simulink model "uC_code"  (R2018b)
settings: Solver=FixedStepDiscrete  StartTime=0.0  StopTime=inf  RelTol=1e-3
PreLoadFcn:
  | LQR_control_design
values from neighbouring files (symbols this model uses):
  ADC_bits = 12    [LQR_control_design.m]    (also in UserSettings.m)
  ADC_Vref = 3.3    [LQR_control_design.m]    (also in UserSettings.m)
  current_gain = 0.5    [LQR_control_design.m]    (also in UserSettings.m)
  current_offset = 1    [LQR_control_design.m]    (also in UserSettings.m)
  K = -K    (= -0.383)    [LQG_control_design.m]    (also in LQR_control_design.m = -(1/R).*B'*Sinf; myLQR.m = -(1/R).*B'*Sinf; myREF.m = [Kw Ki])
  omega_gain = 0.5    [LQR_control_design.m]    (also in UserSettings.m)
  omega_offset = 1    [LQR_control_design.m]    (also in UserSettings.m)
  PPR = 1000    [LQR_control_design.m]    (also in UserSettings.m)
  Vact = 12    [LQR_control_design.m]
undefined symbols (not defined in the file or in its folder): DiscIntNeverNeededParam
libraries: mbedblockslib x5, powerlib_meascontrol x2, dspswit3 x1, discretizing x1
settings Model: ExtModeTrigDuration=10  Creator=angel  LastModifiedBy=angel
settings OptimizationCC: DefaultParameterBehavior=Inlined  UseDivisionForNetSlopeComputation=on  UseFloatMulNetSlope=on  UseSpecifiedMinMax=on  InlineInvariantSignals=on  EnhancedBackFolding=on  BooleansAsBitfields=on  PassReuseOutputArgsAs=Individual arguments  StateBitsets=on  DataBitsets=on  ZeroExternalMemoryAtStartup=off  ZeroInternalMemoryAtStartup=off  NoFixptDivByZeroProtection=on  EfficientFloat2IntCast=on  LifeSpan=1  MaxStackSize=64  OptimizeBlockOrder=speed  DifferentSizesBufferReuse=on
settings DebuggingCC: SignalInfNanChecking=error  IntegerOverflowMsg=error  ParameterTunabilityLossMsg=error  AssertControl=DisableAll  SFUndirectedBroadcastEventsDiag=error
settings HardwareCC: ProdBitPerPointer=32  ProdBitPerSizeT=32  ProdBitPerPtrDiffT=32  ProdLargestAtomicInteger=Long  ProdLargestAtomicFloat=Double  ProdWordSize=32  ProdLongLongMode=on  ProdHWDeviceType=ARM Compatible->ARM Cortex
settings SFSimCC: CompileTimeRecursionLimit=0  EnableRuntimeRecursion=off  MATLABDynamicMemAlloc=off
settings RTWCC: SystemTargetFile=ert.tlc  HardwareBoard=STM32 Nucleo F411RE  TemplateMakefile=ert_default_tmf  GenerateReport=on  Toolchain=GNU Tools for ARM Embedded Processors  BuildConfiguration=Faster Runs  IncludeHyperlinkInReport=on  LaunchReport=on  GenerateTraceInfo=on  GenerateTraceReport=on  GenerateTraceReportSl=on  GenerateTraceReportSf=on  GenerateTraceReportEml=on  GenerateCodeMetricsReport=on
settings CodeAppCC: ForceParamTrailComments=on  IgnoreCustomStorageClasses=off  OperatorAnnotations=on  SimulinkDataObjDesc=on  SFDataObjDesc=on  CustomSymbolStrGlobalVar=rt$N$M  CustomSymbolStrType=$N$M  CustomSymbolStrFcn=$N$M$F  CustomSymbolStrMacro=$N$M  InsertBlockDesc=on
settings ERTTargetCC: UtilityFuncGeneration=Shared location  IncludeMdlTerminateFcn=off  CombineSignalStateStructs=on  SupportAbsoluteTime=off  SupportComplex=off  SupportNonInlinedSFcns=on  ParenthesesLevel=Maximum  CastingMode=Standards  GenerateSharedConstants=off  InlinedParameterPlacement=NonHierarchical  ERTFilePackagingFormat=CompactWithDataFile  EnableSignedLeftShifts=off  EnableSignedRightShifts=off

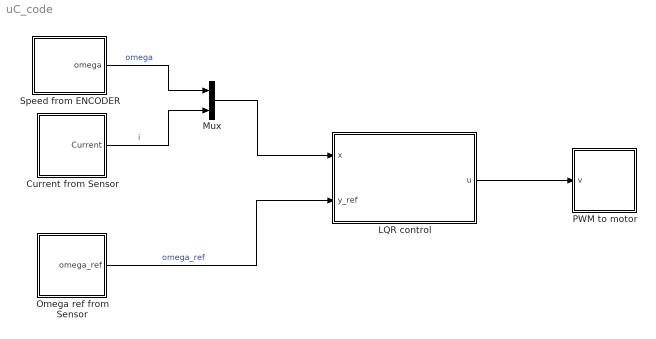
== system uC_code ==
  Current from Sensor : Subsystem
      mask Display: image('E:\Università\Magistrale - Advanced Automotive Electronic Engineering\Compliance Design of Automotive Systems\motor-control\MATLAB\images\lowres-INFIN_Icon_Current_02.eps.png');
  LQR control : Subsystem
  Mux : Mux  Inputs=2
  Omega ref from Sensor : Subsystem
      mask Display: image('E:\Università\Magistrale - Advanced Automotive Electronic Engineering\Compliance Design of Automotive Systems\motor-control\MATLAB\images\65193.png');
  PWM to motor : Subsystem
      mask Display: image('E:\Università\Magistrale - Advanced Automotive Electronic Engineering\Compliance Design of Automotive Systems\motor-control\MATLAB\images\PWM-Icon.png');
  Speed from ENCODER : Subsystem
      mask Display: image('E:\Università\Magistrale - Advanced Automotive Electronic Engineering\Compliance Design of Automotive Systems\motor-control\MATLAB\images\Cattura.JPG');
  wires:
  Speed from ENCODER/1(omega) -> Mux/1  "omega"
  Current from Sensor/1(Current) -> Mux/2  "i"
  Mux/1 -> LQR control/1(x)
  LQR control/1(u) -> PWM to motor/1(v)
  Omega ref from Sensor/1(omega_ref) -> LQR control/2(y_ref)  "omega_ref"

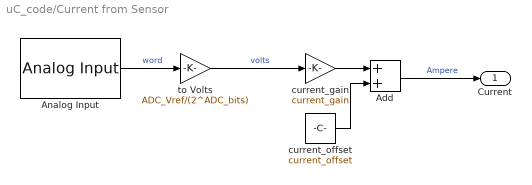
== system uC_code/Current from Sensor ==
  Add : Sum
  Analog Input : mbedblockslib/Analog Input  Pin=PB_0  ReadResultsOnly=off  ConversionTriggerSource=Software  ExternalTriggerType=uint32( 0 )  OutputDataType=double  EnableConversionCompleteNotify=off  EnableOuputStatus=off  SampleTime=-1
      settings: SourceProductName=Simulink Coder Support Package for BBC microbit Board  SourceProductBaseCode=MICROBIT
  current_gain : Gain  Gain=current_gain
  current_offset : Constant  Value=current_offset
  to Volts : Gain  Gain=ADC_Vref/(2^ADC_bits)
  Current : Outport
  wires:
  Analog Input/1 -> to Volts/1  "word"
  current_gain/1 -> Add/1
  current_offset/1 -> Add/2
  to Volts/1 -> current_gain/1  "volts"
  Add/1 -> Current/1  "Ampere"

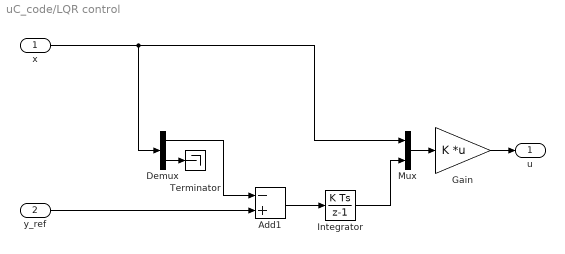
== system uC_code/LQR control ==
  x : Inport
  y_ref : Inport  Port=2
  Add1 : Sum  Inputs=-+
  Demux : Demux  Outputs=2
  Gain : Gain  Gain=K  Multiplication=Matrix(K*u) (u vector)
  Integrator : DiscreteIntegrator  SampleTime=1.0  ICPrevOutput=DiscIntNeverNeededParam  ICPrevScaledInput=DiscIntNeverNeededParam  mask(DiscretizedDiscreteIntegrator){}
      mask init:
      | %zoh
  Mux : Mux  Inputs=2
  Terminator : Terminator
  u : Outport
  wires:
  Mux/1 -> Gain/1
  Demux/1 -> Add1/1
  y_ref/1 -> Add1/2
  Gain/1 -> u/1
  Integrator/1 -> Mux/2
  Add1/1 -> Integrator/1
  x/1 -> Mux/1, Demux/1
  Demux/2 -> Terminator/1

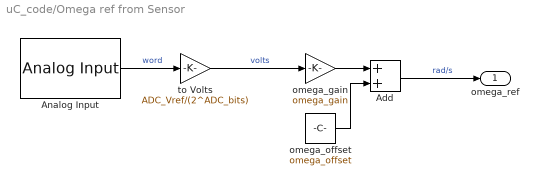
== system uC_code/Omega ref from Sensor ==
  Add : Sum
  Analog Input : mbedblockslib/Analog Input  Pin=PC_0  ReadResultsOnly=off  ConversionTriggerSource=Software  ExternalTriggerType=uint32( 0 )  OutputDataType=double  EnableConversionCompleteNotify=off  EnableOuputStatus=off  SampleTime=-1
      settings: SourceProductName=Simulink Coder Support Package for BBC microbit Board  SourceProductBaseCode=MICROBIT
  omega_gain : Gain  Gain=omega_gain
  omega_offset : Constant  Value=omega_offset
  to Volts : Gain  Gain=ADC_Vref/(2^ADC_bits)
  omega_ref : Outport
  wires:
  Add/1 -> omega_ref/1  "rad/s"
  to Volts/1 -> omega_gain/1  "volts"
  omega_offset/1 -> Add/2
  omega_gain/1 -> Add/1
  Analog Input/1 -> to Volts/1  "word"

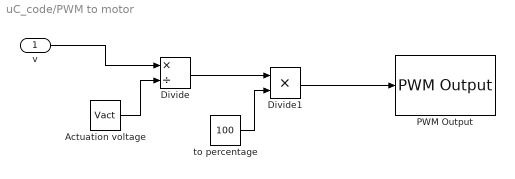
== system uC_code/PWM to motor ==
  v : Inport
  Actuation voltage : Constant  Value=Vact
  Divide : Product  Inputs=*/
  Divide1 : Product  Inputs=**
  PWM Output : mbedblockslib/PWM Output  Pin=PA_3  EnableInputFrequency=off  InitialFrequency=2000  InitialDutyCycle=50  NotificationType=None
      settings: SourceProductName=Simulink Coder Support Package for BBC microbit Board  SourceProductBaseCode=MICROBIT
  to percentage : Constant  Value=100
  wires:
  Actuation voltage/1 -> Divide/2
  v/1 -> Divide/1
  Divide/1 -> Divide1/1
  to percentage/1 -> Divide1/2
  Divide1/1 -> PWM Output/1

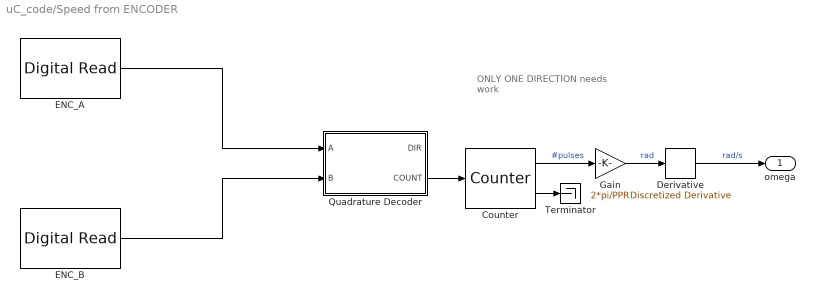
== system uC_code/Speed from ENCODER ==
  note: ONLY ONE DIRECTION
      | needs work
  Counter : dspswit3/Counter  Direction=Up  CountEvent=Rising edge  CounterSize=User defined  MaxCount=255  InitialCount=0  Output=Count and Hit  HitValue=32  ResetInput=off  SamplesPerFrame=1  Ts=1  CntDtype=double  HitDtype=Logical
  Derivative : discretizing/Discretized Derivative  method=tustin  SampleTime=1.0  Wc=1
  ENC_A : mbedblockslib/Digital Read  Pin=PA_0  Direction=input  SampleTime=-1
      settings: SourceProductName=Simulink Coder Support Package for BBC microbit Board  SourceProductBaseCode=MICROBIT
  ENC_B : mbedblockslib/Digital Read  Pin=PA_1  Direction=input  SampleTime=-1
      settings: SourceProductName=Simulink Coder Support Package for BBC microbit Board  SourceProductBaseCode=MICROBIT
  Gain : Gain  Gain=2*pi/PPR
  Quadrature Decoder : Subsystem
  Terminator : Terminator
  omega : Outport
  wires:
  ENC_A/1 -> Quadrature Decoder/1(A)
  ENC_B/1 -> Quadrature Decoder/2(B)
  Quadrature Decoder/2(COUNT) -> Counter/1
  Counter/1 -> Gain/1  "#pulses"
  Gain/1 -> Derivative/1  "rad"
  Derivative/1 -> omega/1  "rad/s"
  Counter/2 -> Terminator/1

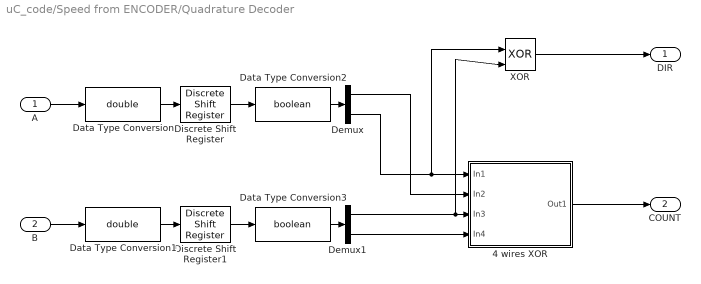
== system uC_code/Speed from ENCODER/Quadrature Decoder ==
  A : Inport
  B : Inport  Port=2
  4 wires XOR : Subsystem
  Data Type Conversion : DataTypeConversion  OutDataTypeStr=double
  Data Type Conversion1 : DataTypeConversion  OutDataTypeStr=double
  Data Type Conversion2 : DataTypeConversion  OutDataTypeStr=boolean
  Data Type Conversion3 : DataTypeConversion  OutDataTypeStr=boolean
  Demux : Demux  Outputs=2
  Demux1 : Demux  Outputs=2
  Discrete Shift Register : powerlib_meascontrol/Additional Components/Discrete Shift Register  NSamples=2  InitialValue=0  Ts=50e-6
      settings: SourceProductName=Simscape Power Systems  SourceProductBaseCode=PS
  Discrete Shift Register1 : powerlib_meascontrol/Additional Components/Discrete Shift Register  NSamples=2  InitialValue=0  Ts=50e-6
      settings: SourceProductName=Simscape Power Systems  SourceProductBaseCode=PS
  XOR : Logic  Operator=XOR  IconShape=distinctive  AllPortsSameDT=off  OutDataTypeStr=boolean
  DIR : Outport
  COUNT : Outport  Port=2
  wires:
  4 wires XOR/1(Out1) -> COUNT/1
  Demux/1 -> 4 wires XOR/2(In2)
  Demux/2 -> XOR/1, 4 wires XOR/1(In1)
  Demux1/1 -> XOR/2, 4 wires XOR/3(In3)
  Demux1/2 -> 4 wires XOR/4(In4)
  XOR/1 -> DIR/1
  A/1 -> Data Type Conversion/1
  Data Type Conversion/1 -> Discrete Shift Register/1
  Data Type Conversion1/1 -> Discrete Shift Register1/1
  B/1 -> Data Type Conversion1/1
  Discrete Shift Register/1 -> Data Type Conversion2/1
  Data Type Conversion2/1 -> Demux/1
  Discrete Shift Register1/1 -> Data Type Conversion3/1
  Data Type Conversion3/1 -> Demux1/1

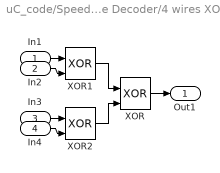
== system uC_code/Speed from ENCODER/Quadrature Decoder/4 wires XOR ==
  In1 : Inport
  In2 : Inport  Port=2
  In3 : Inport  Port=3
  In4 : Inport  Port=4
  XOR : Logic  Operator=XOR  IconShape=distinctive  AllPortsSameDT=off  OutDataTypeStr=boolean
  XOR1 : Logic  Operator=XOR  IconShape=distinctive  AllPortsSameDT=off  OutDataTypeStr=boolean
  XOR2 : Logic  Operator=XOR  IconShape=distinctive  AllPortsSameDT=off  OutDataTypeStr=boolean
  Out1 : Outport
  wires:
  In1/1 -> XOR1/1
  XOR2/1 -> XOR/2
  XOR1/1 -> XOR/1
  XOR/1 -> Out1/1
  In3/1 -> XOR2/1
  In2/1 -> XOR1/2
  In4/1 -> XOR2/2
